simulink model "motion_example1"  (Simulink 10.0)
settings: Solver=ode45  StartTime=0.0  StopTime=3  EnableMultiTasking=on
libraries: motion x2
settings Model: Creator=bhisma  LastModifiedBy=bhisma  ExtModeTrigMode=oneshot  ExtModeArmWhenConnect=off
settings DataIOCC: SignalLoggingSaveFormat=ModelDataLogs
settings OptimizationCC: BooleanDataType=off  LifeSpan=auto
settings DebuggingCC: SaveWithParameterizedLinksMsg=none  SignalResolutionControl=TryResolveAllWithWarning  MultiTaskDSMMsg=warning  MultiTaskCondExecSysMsg=none  SFUnexpectedBacktrackingDiag=error  SFNoUnconditionalDefaultTransitionDiag=error  SFExecutionAtInitializationDiag=warning  ArithmeticOperatorsInVariantConditions=error
settings HardwareCC: ProdBitPerPointer=64  ProdBitPerSizeT=64  ProdBitPerPtrDiffT=64  ProdLargestAtomicFloat=Float  ProdIntDivRoundTo=Zero  ProdEndianess=LittleEndian  ProdWordSize=64  ProdHWDeviceType=Intel->x86-64 (Windows64)  TargetUnknown=on
settings SFSimCC: SimUseLocalCustomCode=on  CustomCodeUndefinedFunction=FilterOut
settings RTWCC: RTWUseLocalCustomCode=on
settings CodeAppCC: StateflowObjectComments=off
settings GRTTargetCC: TargetLangStandard=C99 (ISO)
settings ConfigComp: CovMetricSettings=dwe  CovSaveCumulativeToWorkspaceVar=off  CovSaveSingleToWorkspaceVar=off

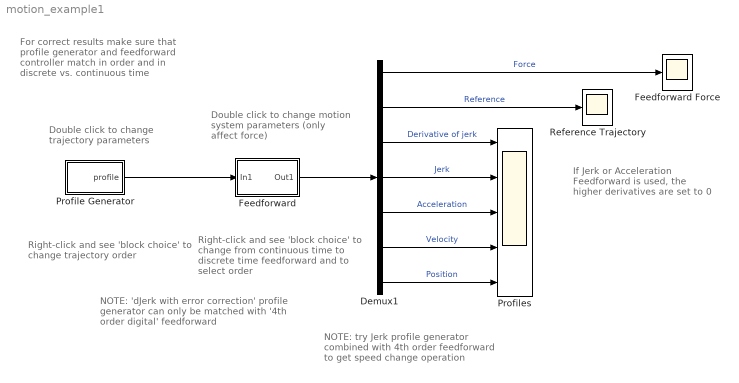
== system motion_example1 ==
  note: Double click to change
      | trajectory parameters
  note: Double click to change
      | motion system parameters
      | (only affect force)
  note: Right-click and see 'block choice'
      | to change from continuous time
      | to discrete time feedforward and
      | to select order
  note: For correct results make sure that
      | profile generator and feedforward
      | controller match in order and in
      | discrete vs. continuous time
  note: Right-click and see 'block choice'
      | to change trajectory order
  note: NOTE: 'dJerk with error correction'
      | profile generator can only be matched
      | with '4th order digital' feedforward
  note: If Jerk or Acceleration
      | Feedforward is used,
      | the higher derivatives
      | are set to 0
  note: NOTE: try Jerk profile generator
      | combined with 4th order feedforward
      | to get speed change operation
  Demux1 : Demux  Outputs=7
  Feedforward : Subsystem  BlockChoice=4th order continuous
      link override 2nd order discrete: Ts=1e-1
      link override 3d order continuous: q2=0
      link override 3d order discrete: Ts=1e-1
      link override 4th order continuous: m1=20  c=6e5
      link override 4th order digital: Ts=1e-3
      link override 4th order discrete: Ts=1e-2
      settings: AttributesFormatString=%<BlockChoice>  TemplateBlock=motion/Feedforward Controllers/Feedforward  MemberBlocks=2nd order continuous,2nd order discrete,3d order continuous,3d order discrete,4th order continuous,4th order digital,4th order discrete
  Feedforward Force : Scope
  Profile Generator : Subsystem  BlockChoice=Derivative of Jerk
      link override Acceleration: Ts=1e-1  a=5
      link override Derivative of Jerk: Ts=1e-2
      link override Jerk: Ts=0
      link override dJerk with error correction: Ts=1e-3
      settings: AttributesFormatString=%<BlockChoice>  TemplateBlock=motion/Profile Generators/Profile Generator  MemberBlocks=Acceleration,Derivative of Jerk,Jerk,dJerk with error correction
  Profiles : Scope  NumInputPorts=5
  Reference Trajectory : Scope
  wires:
  Feedforward/1(Out1) -> Demux1/1
  Demux1/1 -> Feedforward Force/1  "Force"
  Demux1/2 -> Reference Trajectory/1  "Reference"
  Demux1/3 -> Profiles/1  "Derivative of jerk"
  Demux1/4 -> Profiles/2  "Jerk"
  Demux1/5 -> Profiles/3  "Acceleration"
  Demux1/6 -> Profiles/4  "Velocity"
  Demux1/7 -> Profiles/5  "Position"
  Profile Generator/1(profile) -> Feedforward/1(In1)

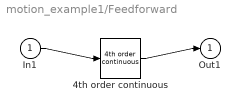
== system motion_example1/Feedforward ==
  In1 : Inport
  4th order continuous : motion/Feedforward Controllers/4th order continuous  m1=20  m2=10  k1=10  k2=10  c=6e5  k12=500
  Out1 : Outport
  wires:
  In1/1 -> 4th order continuous/1
  4th order continuous/1 -> Out1/1

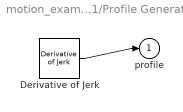
== system motion_example1/Profile Generator ==
  Derivative of Jerk : motion/Profile Generators/Derivative of Jerk  t0=.3  x=1  v=1  a=5  j=50  d=1000  Ts=1e-2
  profile : Outport
  wires:
  Derivative of Jerk/1 -> profile/1
